simulink model "BHclientP"  (Simulink 7.4)
settings: Solver=ode3  StartTime=0.0  StopTime=inf  FixedStep=0.005  RelTol=1e-3
libraries: planmant x1
settings Model: Creator=Admin  LastModifiedBy=Admin

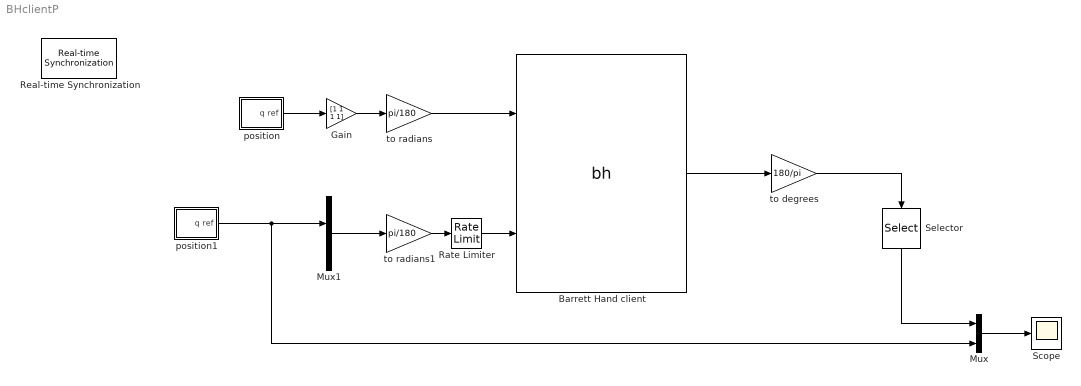
== system BHclientP ==
  Barrett Hand client : S-Function  FunctionName=bh  Parameters=IP port mode262 mode280 ST a0 a1 a2 a3 a4 a41 a5 a6 a7 a8 a81 a9  EnableBusSupport=off  mask(Barrett Hand UDP client){mode262=Position, mode280=Position, IP=193.2.6.168, port=4444, ST=0.005, a0=off, a1=off, a2=off, a3=off, a4=off, a41=off, a5=on, a6=off, a7=off, a8=off, a81=off, a9=off}
      mask prompts: mode262 "BH262 mode"; mode280 "BH280 mode"; port "UDP port"; a0 "Time"; a1 "262 position"; a2 "262 velocity"; a3 "262 deltap"; a4 "262 strain"; a41 "262 strain filt"; a5 "280 position"; a6 "280 velocity"; a7 "280 deltap"; a8 "280 strain"; a81 "280 strain filt"; a9 "pps"
      mask help:
      | Make sure you select the right mode. Sending positions when velocity mode
      | selected may not end well.
      |
      | Units are rad and rad/s. Strain and pps data is raw (no units)
      mask StyleString: popup(Velocity|Position|Torque|Other),popup(Velocity|Position|Torque|Other),edit,edit,edit,checkbox,checkbox,checkbox,checkbox,checkbox,checkbox,checkbox,checkbox,checkbox,checkbox,checkbox,checkbox
      mask CallbackString: togglePorts()|togglePorts()|togglePorts()|togglePorts()||togglePorts()|togglePorts()|togglePorts()|togglePorts()|togglePorts()|togglePorts()|togglePorts()|togglePorts()|togglePorts()|togglePorts()|togglePorts()|togglePorts()
      mask TabNameString: Control,Control,Control,Control,Control,Outputs,Outputs,Outputs,Outputs,Outputs,Outputs,Outputs,Outputs,Outputs,Outputs,Outputs,Outputs
      mask Display: text(0.3, 0.9, '\fontsize{10}IP: {\bf193.2.6.168 \newline\rmport: \bf4444}', 'horizontalAlignment', 'center','texmode','on')color('blue') port_label('input',1,'\fontsize{12}BH262 {\newline\bfPosition}','texmode','on')color('blue') port_label('input',2,'\fontsize{12}BH280 {\newline\bfPosition}','texmode','on')color('black')port_label('output',1,'\fontsize{11}BH280 {\bfPosition}','texmode','on');
  Gain : Gain  Gain=[1 1 1 1]  ParameterDataType=fixdt(1, 16)  ParameterScaling=2^0  OutDataType=fixdt(1, 16)  OutScaling=2^0
  Mux : Mux  Inputs=2
  Mux1 : Mux
  Rate Limiter : RateLimiter  RisingSlewLimit=0.5  FallingSlewLimit=-0.5  SampleTimeMode=inherited
  Real-time Synchronization : planmant/Utility/Real-time Synchronization  SystemSampleTime=-1
  Scope : Scope
      settings: YMin=0  YMax=90
  Selector : Selector  InputPortWidth=4  IndexOptions=Index vector (dialog)  Indices=2  OutputSizes=1
  position : Subsystem
  position1 : Subsystem
  to degrees : Gain  Gain=180/pi  ParameterDataType=fixdt(1, 16)  ParameterScaling=2^0  OutDataType=fixdt(1, 16)  OutScaling=2^0
  to radians : Gain  Gain=pi/180  ParameterDataType=fixdt(1, 16)  ParameterScaling=2^0  OutDataType=fixdt(1, 16)  OutScaling=2^0
  to radians1 : Gain  Gain=pi/180  ParameterDataType=fixdt(1, 16)  ParameterScaling=2^0  OutDataType=fixdt(1, 16)  OutScaling=2^0
  wires:
  Mux/1 -> Scope/1
  Gain/1 -> to radians/1
  position/1(q ref) -> Gain/1
  to degrees/1 -> Selector/1
  position1/1(q ref) -> Mux/2, Mux1/2
  to radians/1 -> Barrett Hand client/1
  Barrett Hand client/1 -> to degrees/1
  Rate Limiter/1 -> Barrett Hand client/2
  Mux1/1 -> to radians1/1
  to radians1/1 -> Rate Limiter/1
  Selector/1 -> Mux/1

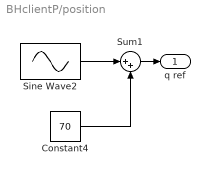
== system BHclientP/position ==
  Constant4 : Constant  Value=70  OutDataType=fixdt(1, 16)  OutScaling=2^0
  Sine Wave2 : Sin  Amplitude=30  Bias=0  Frequency=pi  Phase=pi/4  Samples=10  Offset=0
  Sum1 : Sum  Inputs=|++  OutDataType=fixdt(1, 16)  OutScaling=2^0
  q ref : Outport
  wires:
  Sine Wave2/1 -> Sum1/1
  Constant4/1 -> Sum1/2
  Sum1/1 -> q ref/1

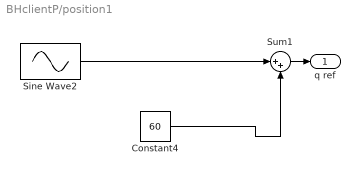
== system BHclientP/position1 ==
  Constant4 : Constant  Value=60  OutDataType=fixdt(1, 16)  OutScaling=2^0
  Sine Wave2 : Sin  Amplitude=30  Bias=0  Frequency=0.1*pi  Phase=pi/4  Samples=10  Offset=0
  Sum1 : Sum  Inputs=|++  OutDataType=fixdt(1, 16)  OutScaling=2^0
  q ref : Outport
  wires:
  Constant4/1 -> Sum1/2
  Sum1/1 -> q ref/1
  Sine Wave2/1 -> Sum1/1
